simulink model "octocopter_model_test"  (R2023a)
settings: Solver=VariableStepAuto  StartTime=0.0  StopTime=10.0  RelTol=1e-3
values from neighbouring files (symbols this model uses):
  k_M = 8e-5    (= 8e-05)    [drone_data.m]
  k_T = 3e-4    (= 0.0003)    [drone_data.m]
  l = 0.22414    [drone_data.m]
  lxx = 3.426e-5    (= 3.426e-05)    [drone_data.m]
  lyy = 2.00298e-3    (= 0.00200298)    [drone_data.m]
  lzz = 2.01834e-3    (= 0.00201834)    [drone_data.m]
  m = 0.7227    [drone_data.m]
  U = wh * ones(8, 1)    [octocopter_model_test_script.m]
  X0 = zeros(12, 1)    [octocopter_model_test_script.m]
undefined symbols (not defined in the file or in its folder): octocopter_kinematics
settings Model: Creator=mluser  LastModifiedBy=mluser

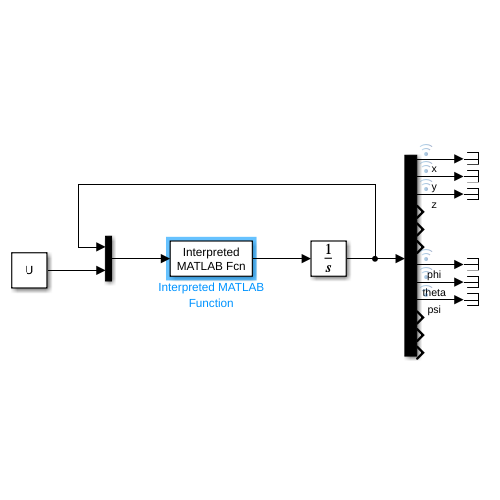
[thumbnail: Simulink's stored preview of the top-level diagram]
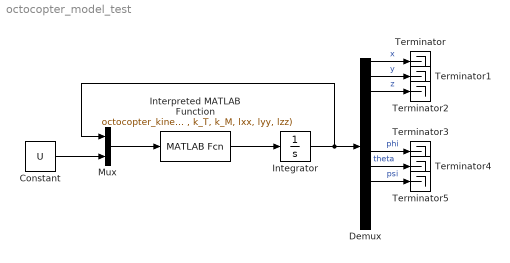
== system octocopter_model_test ==
  Constant : Constant  Value=U
  Demux : Demux  Outputs=12
  Integrator : Integrator  InitialCondition=X0
  Interpreted MATLAB Function : MATLABFcn  MATLABFcn=octocopter_kinematics(u(1:12), u(13:20), m, l , k_T, k_M, lxx, lyy, lzz)
  Mux : Mux  Inputs=2
  Terminator{,1..5} (6 alike) : Terminator
  wires:
  Mux/1 -> Interpreted MATLAB Function/1
  Demux/7 -> Terminator3/1  "phi"
  Integrator/1 -> Mux/1, Demux/1
  Constant/1 -> Mux/2
  Interpreted MATLAB Function/1 -> Integrator/1
  Demux/1 -> Terminator/1  "x"
  Demux/2 -> Terminator1/1  "y"
  Demux/9 -> Terminator5/1  "psi"
  Demux/8 -> Terminator4/1  "theta"
  Demux/3 -> Terminator2/1  "z"
